simulink model "35 Bus Network Electricity Transmission Model"  (R2023b)
settings: Solver=VariableStepAuto  StartTime=0.0  StopTime=1  RelTol=1e-3
model workspace (MAT data in the model file):
  T_set = 0.0001
  Tp = 5e-05
undefined symbols (not defined in the file): D1, D11, Delta, DiscIntNeverNeededParam
libraries: spsSeriesRLCBranchLib x57, spsLoadFlowBusLib x35, spsThreePhaseSeriesRLCLoadLib x28, spsThreePhaseTransformerTwoWindingsLib x22, spsDistributedParametersLineLib x22, spsGenericPowerSystemStabilizerLib x20, spsThreePhaseVIMeasurementLib x14, spsSynchronousMachinepuStandardLib x10, spsExcitationSystemLib x10, spsHydraulicTurbineandGovernorLib x10, spsFourierLib x8, spsMeanLib x8
(part 6 of 8)

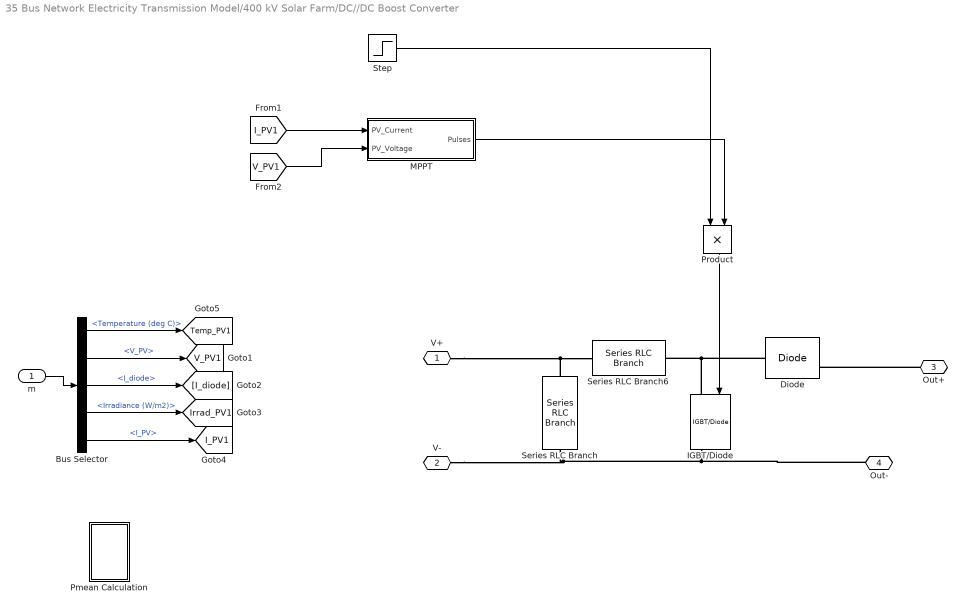
== system 35 Bus Network Electricity Transmission Model/400 kV Solar Farm/DC//DC Boost Converter ==
  m : Inport
  Bus Selector : BusSelector  OutputSignals=Temperature (deg C),V_PV,I_diode,Irradiance (W/m2),I_PV
  Diode : spsDiodeLib/Diode  Ron=0.0001  Lon=0  Vf=0.8  IC=0  UseSnubber=0  Rs=500  Cs=250e-9  Measurements=on
  IGBT/Diode : spsIGBTDiodeLib/IGBT//Diode  Ron=1e-3  Rs=1e5  Cs=inf  Measurements=on
  MPPT : Subsystem  mask{fp=5000, MPPT_time=2e-4, Di=0.62}
      mask prompts: fp "PWM Frequency"; MPPT_time "Time duration for MPPT"; Di "Initialization for Duty Cycle"
  Pmean Calculation : Subsystem
  Product : Product
  Series RLC Branch : spsSeriesRLCBranchLib/Series RLC Branch  LConnTagsString=__new0  RConnTagsString=__new0  BranchType=C  Resistance=1  Inductance=1e-3  SetiL0=off  InitialCurrent=0  Capacitance=1e-4  Setx0=off  InitialVoltage=0  Measurements=None
  Series RLC Branch6 : spsSeriesRLCBranchLib/Series RLC Branch  LConnTagsString=__new0  RConnTagsString=__new0  BranchType=RL  Resistance=0.005  Inductance=5e-3  SetiL0=off  InitialCurrent=0  Capacitance=0  Setx0=off  InitialVoltage=0  Measurements=None
  Step : Step  Time=0.02  SampleTime=0
  V+ : PMIOPort  Side=Left
  V- : PMIOPort  Port=2  Side=Left
  Out+ : PMIOPort  Port=3  Side=Right
  Out- : PMIOPort  Port=4  Side=Right
  tag scope: I_PV1=global, Irrad_PV1=global, Temp_PV1=global, V_PV1=global
  wires:
  [I_PV1] -> MPPT/1(PV_Current)
  Bus Selector/3 -> [I_diode]  "<I_diode>"
  m/1 -> Bus Selector/1
  Bus Selector/5 -> [I_PV1]  "<I_PV>"
  Bus Selector/1 -> [Temp_PV1]  "<Temperature (deg C)>"
  Bus Selector/2 -> [V_PV1]  "<V_PV>"
  [V_PV1] -> MPPT/2(PV_Voltage)
  Step/1 -> Product/1
  MPPT/1(Pulses) -> Product/2
  Product/1 -> IGBT/Diode/1
  Bus Selector/4 -> [Irrad_PV1]  "<Irradiance (W/m2)>"
  connections:
  Series RLC Branch/LConn1 -- V+/RConn1 -- Series RLC Branch6/LConn1
  IGBT/Diode/LConn1 -- Diode/LConn1 -- Series RLC Branch6/RConn1
  IGBT/Diode/RConn1 -- Out-/RConn1 -- V-/RConn1 -- Series RLC Branch/RConn1
  Out+/RConn1 -- Diode/RConn1

== system 35 Bus Network Electricity Transmission Model/400 kV Solar Farm/DC//DC Boost Converter1 ==
  m : Inport
  Bus Selector : BusSelector  OutputSignals=Temperature (deg C),V_PV,I_diode,Irradiance (W/m2),I_PV
  Deblock Converter : Step  Time=0.02  SampleTime=0
  Diode : spsDiodeLib/Diode  Ron=0.0001  Lon=0  Vf=0.8  IC=0  UseSnubber=0  Rs=inf  Cs=inf  Measurements=on
  IGBT/Diode : spsIGBTDiodeLib/IGBT//Diode  Ron=1e-3  Rs=1e5  Cs=inf  Measurements=on
  MPPT : Subsystem  mask{fp=5000, MPPT_time=2e-4, Di=0.62}
      mask prompts: fp "PWM Frequency"; MPPT_time "Time duration for MPPT"; Di "Initialization for Duty Cycle"
  Pmean Calculation : Subsystem
  Product : Product
  Series RLC Branch : spsSeriesRLCBranchLib/Series RLC Branch  LConnTagsString=__new0  RConnTagsString=__new0  BranchType=C  Resistance=1  Inductance=1e-3  SetiL0=off  InitialCurrent=0  Capacitance=1e-4  Setx0=off  InitialVoltage=0  Measurements=None
  Series RLC Branch6 : spsSeriesRLCBranchLib/Series RLC Branch  LConnTagsString=__new0  RConnTagsString=__new0  BranchType=RL  Resistance=0.005  Inductance=5e-3  SetiL0=off  InitialCurrent=0  Capacitance=0  Setx0=off  InitialVoltage=0  Measurements=None
  V+ : PMIOPort  Side=Left
  V- : PMIOPort  Port=2  Side=Left
  Out+ : PMIOPort  Port=3  Side=Right
  Out- : PMIOPort  Port=4  Side=Right
  tag scope: I_PV2=global, Irrad_PV2=global, Temp_PV2=global, V_PV2=global
  wires:
  [I_PV2] -> MPPT/1(PV_Current)
  Bus Selector/3 -> [I_diode]  "<I_diode>"
  m/1 -> Bus Selector/1
  Bus Selector/5 -> [I_PV2]  "<I_PV>"
  Bus Selector/1 -> [Temp_PV2]  "<Temperature (deg C)>"
  Bus Selector/2 -> [V_PV2]  "<V_PV>"
  Bus Selector/4 -> [Irrad_PV2]  "<Irradiance (W/m2)>"
  [V_PV2] -> MPPT/2(PV_Voltage)
  MPPT/1(Pulses) -> Product/1
  Deblock Converter/1 -> Product/2
  Product/1 -> IGBT/Diode/1
  connections:
  Series RLC Branch6/LConn1 -- Series RLC Branch/LConn1 -- V+/RConn1
  IGBT/Diode/LConn1 -- Diode/LConn1 -- Series RLC Branch6/RConn1
  V-/RConn1 -- Series RLC Branch/RConn1 -- IGBT/Diode/RConn1 -- Out-/RConn1
  Out+/RConn1 -- Diode/RConn1

== system 35 Bus Network Electricity Transmission Model/400 kV Solar Farm/DC//DC Boost Converter2 ==
  m : Inport
  Bus Selector : BusSelector  OutputSignals=Temperature (deg C),V_PV,I_diode,Irradiance (W/m2),I_PV
  Diode : spsDiodeLib/Diode  Ron=0.0001  Lon=0  Vf=0.8  IC=0  UseSnubber=0  Rs=inf  Cs=inf  Measurements=on
  IGBT/Diode : spsIGBTDiodeLib/IGBT//Diode  Ron=1e-3  Rs=1e5  Cs=inf  Measurements=on
  MPPT : Subsystem  mask{fp=5000, MPPT_time=2e-4, Di=0.62}
      mask prompts: fp "PWM Frequency"; MPPT_time "Time duration for MPPT"; Di "Initialization for Duty Cycle"
  Pmean Calculation : Subsystem
  Product : Product
  Series RLC Branch : spsSeriesRLCBranchLib/Series RLC Branch  LConnTagsString=__new0  RConnTagsString=__new0  BranchType=C  Resistance=1  Inductance=1e-3  SetiL0=off  InitialCurrent=0  Capacitance=1e-4  Setx0=off  InitialVoltage=0  Measurements=None
  Series RLC Branch6 : spsSeriesRLCBranchLib/Series RLC Branch  LConnTagsString=__new0  RConnTagsString=__new0  BranchType=RL  Resistance=0.005  Inductance=5e-3  SetiL0=off  InitialCurrent=0  Capacitance=0  Setx0=off  InitialVoltage=0  Measurements=None
  Step : Step  Time=0.02  SampleTime=0
  V+ : PMIOPort  Side=Left
  V- : PMIOPort  Port=2  Side=Left
  Out+ : PMIOPort  Port=3  Side=Right
  Out- : PMIOPort  Port=4  Side=Right
  tag scope: I_PV3=global, Irrad_PV3=global, Temp_PV3=global, V_PV3=global
  wires:
  [I_PV3] -> MPPT/1(PV_Current)
  Bus Selector/3 -> [I_diode]  "<I_diode>"
  m/1 -> Bus Selector/1
  Bus Selector/5 -> [I_PV3]  "<I_PV>"
  Bus Selector/1 -> [Temp_PV3]  "<Temperature (deg C)>"
  Bus Selector/2 -> [V_PV3]  "<V_PV>"
  Bus Selector/4 -> [Irrad_PV3]  "<Irradiance (W/m2)>"
  [V_PV3] -> MPPT/2(PV_Voltage)
  Step/1 -> Product/2
  MPPT/1(Pulses) -> Product/1
  Product/1 -> IGBT/Diode/1
  connections:
  Series RLC Branch6/LConn1 -- Series RLC Branch/LConn1 -- V+/RConn1
  IGBT/Diode/LConn1 -- Diode/LConn1 -- Series RLC Branch6/RConn1
  V-/RConn1 -- Series RLC Branch/RConn1 -- IGBT/Diode/RConn1 -- Out-/RConn1
  Out+/RConn1 -- Diode/RConn1

== system 35 Bus Network Electricity Transmission Model/400 kV Solar Farm/DC//DC Boost Converter3 ==
  m : Inport
  Bus Selector : BusSelector  OutputSignals=Temperature (deg C),V_PV,I_diode,Irradiance (W/m2),I_PV
  Diode : spsDiodeLib/Diode  Ron=0.0001  Lon=0  Vf=0.8  IC=0  UseSnubber=0  Rs=inf  Cs=inf  Measurements=on
  IGBT/Diode : spsIGBTDiodeLib/IGBT//Diode  Ron=1e-3  Rs=1e5  Cs=inf  Measurements=on
  MPPT : Subsystem  mask{fp=5000, MPPT_time=2e-4, Di=0.62}
      mask prompts: fp "PWM Frequency"; MPPT_time "Time duration for MPPT"; Di "Initialization for Duty Cycle"
  Pmean Calculation : Subsystem
  Product : Product
  Series RLC Branch : spsSeriesRLCBranchLib/Series RLC Branch  LConnTagsString=__new0  RConnTagsString=__new0  BranchType=C  Resistance=1  Inductance=1e-3  SetiL0=off  InitialCurrent=0  Capacitance=1e-4  Setx0=off  InitialVoltage=0  Measurements=None
  Series RLC Branch6 : spsSeriesRLCBranchLib/Series RLC Branch  LConnTagsString=__new0  RConnTagsString=__new0  BranchType=RL  Resistance=0.005  Inductance=5e-3  SetiL0=off  InitialCurrent=0  Capacitance=0  Setx0=off  InitialVoltage=0  Measurements=None
  Step : Step  Time=0.02  SampleTime=0
  V+ : PMIOPort  Side=Left
  V- : PMIOPort  Port=2  Side=Left
  Out+ : PMIOPort  Port=3  Side=Right
  Out- : PMIOPort  Port=4  Side=Right
  tag scope: I_PV4=global, Irrad_PV4=global, Temp_PV4=global, V_PV4=global
  wires:
  [I_PV4] -> MPPT/1(PV_Current)
  Bus Selector/3 -> [I_diode]  "<I_diode>"
  m/1 -> Bus Selector/1
  Bus Selector/5 -> [I_PV4]  "<I_PV>"
  Bus Selector/1 -> [Temp_PV4]  "<Temperature (deg C)>"
  Bus Selector/2 -> [V_PV4]  "<V_PV>"
  [V_PV4] -> MPPT/2(PV_Voltage)
  Step/1 -> Product/2
  MPPT/1(Pulses) -> Product/1
  Product/1 -> IGBT/Diode/1
  Bus Selector/4 -> [Irrad_PV4]  "<Irradiance (W/m2)>"
  connections:
  Series RLC Branch6/LConn1 -- Series RLC Branch/LConn1 -- V+/RConn1
  IGBT/Diode/LConn1 -- Diode/LConn1 -- Series RLC Branch6/RConn1
  V-/RConn1 -- Series RLC Branch/RConn1 -- IGBT/Diode/RConn1 -- Out-/RConn1
  Out+/RConn1 -- Diode/RConn1

== system 35 Bus Network Electricity Transmission Model/400 kV Solar Farm/VSC Control ==
  Vabc_prim : Inport  PortDimensions=3
  Iabc_prim : Inport  Port=2  PortDimensions=3
  Vdc_mes : Inport  Port=3  PortDimensions=1
  Current Regulator : Subsystem
  Iq_ref : Constant  Value=0
  Mux : Mux  Inputs=2
  PLL & Measurements : Subsystem
  PWM Generator (3-Level) : spsPWMGenerator3LevelLib/PWM Generator (3-Level)  ModulatorType=Three-phase bridge (12 pulses)  ModulatorMode=Unsynchronized  nF=27  Fc=33*60  ModulatingSignals=off  m=0.8  Freq=60  Phase=0  Ts=5e-5
  Uabc_ref Generation max (m) = 1 : Subsystem
  Unit Delay : UnitDelay  SampleTime=T_set  HasFrameUpgradeWarning=on
  VDC Regulator : Subsystem
  Vdc_ref1 : Constant  Value=Vdc_ref
  Pulses : Outport  VectorParamsAs1DForOutWhenUnconnected=off
  wires:
  VDC Regulator/1(Id_ref) -> Mux/1
  PLL & Measurements/1(wt) -> Uabc_ref Generation max (m) = 1/1(wt)
  Current Regulator/1(VdVq_conv) -> Uabc_ref Generation max (m) = 1/2(VdVq_conv)
  Iq_ref/1 -> Mux/2
  Mux/1 -> Current Regulator/3(IdIq_ref)
  PLL & Measurements/3(IdIq_prim) -> Current Regulator/2(IdIq_mes)
  PLL & Measurements/2(VdVq_prim) -> Current Regulator/1(VdVq_mes)
  Vdc_mes/1 -> VDC Regulator/1(Vdc_mes)
  Vabc_prim/1 -> PLL & Measurements/1(Vabc_prim)
  Iabc_prim/1 -> PLL & Measurements/2(Iabc_prim)
  Unit Delay/1 -> PWM Generator (3-Level)/1
  PWM Generator (3-Level)/1 -> Pulses/1
  Uabc_ref Generation max (m) = 1/1(Uabc_ref) -> Unit Delay/1
  Vdc_ref1/1 -> VDC Regulator/2(Vdc_ref)

== system 35 Bus Network Electricity Transmission Model/Home Network Load （with circuit breaker)/Circuit Breaker ==
  "Reset " : Inport
  Abs : Abs  SaturateOnIntegerOverflow=off
  Current Measurement1 : spsCurrentMeasurementLib/Current Measurement  PhasorSimulation=off  OutputType=Complex  PSBequivalent=0
  Data Type Conversion : DataTypeConversion  OutDataTypeStr=boolean  SaturateOnIntegerOverflow=off  RndMeth=Floor
  Data Type Conversion1 : DataTypeConversion  OutDataTypeStr=double  SaturateOnIntegerOverflow=off  RndMeth=Floor
  Hit Crossing : HitCross
  Ideal Switch : spsIdealSwitchLib/Ideal Switch  Ron=0.01  Lon=0  IC=0  Rs=1e5  Cs=inf  Measurements=on
  Logical Operator : Logic  AllPortsSameDT=off  OutDataTypeStr=boolean
  Relational Operator : RelationalOperator  Operator=<=  OutDataTypeStr=boolean  RndMeth=Simplest  InputSameDT=off
  S-R Flip-Flop : simulink_extras/Flip Flops/S-R Flip-Flop  initial_condition=0
  S-R Flip-Flop1 : simulink_extras/Flip Flops/S-R Flip-Flop  initial_condition=0
  Static Trip Current : Constant  Value=110
  Terminator : Terminator
  Terminator1 : Terminator
  Terminator2 : Terminator
  Transfer Fcn : TransferFcn  Denominator=[0.001 1]
  Connection Port1 : PMIOPort  Side=Left
  Connection Port : PMIOPort  Port=2  Side=Right
  wires:
  Logical Operator/1 -> S-R Flip-Flop1/2
  Current Measurement1/1 -> Hit Crossing/1, Abs/1
  Hit Crossing/1 -> Logical Operator/2
  Transfer Fcn/1 -> Relational Operator/1
  S-R Flip-Flop1/2 -> Terminator1/1
  Ideal Switch/1 -> Terminator2/1
  S-R Flip-Flop/1 -> Logical Operator/1
  Abs/1 -> Transfer Fcn/1
  "Reset "/1 -> Data Type Conversion/1
  S-R Flip-Flop1/1 -> Data Type Conversion1/1
  Relational Operator/1 -> S-R Flip-Flop/1
  Data Type Conversion/1 -> S-R Flip-Flop/2, S-R Flip-Flop1/1
  S-R Flip-Flop/2 -> Terminator/1
  Data Type Conversion1/1 -> Ideal Switch/1
  Static Trip Current/1 -> Relational Operator/2
  connections:
  Connection Port1/RConn1 -- Ideal Switch/LConn1
  Current Measurement1/LConn1 -- Ideal Switch/RConn1
  Connection Port/RConn1 -- Current Measurement1/RConn1

== system 35 Bus Network Electricity Transmission Model/North Network/Cs BMW- MPP8 ==
  Series RLC Branch : spsSeriesRLCBranchLib/Series RLC Branch  LConnTagsString=__new0  RConnTagsString=__new0  BranchType=C  Resistance=1  Inductance=1e-3  SetiL0=off  InitialCurrent=0  Capacitance=0.00049736  Setx0=off  InitialVoltage=0  Measurements=None
  Series RLC Branch1 : spsSeriesRLCBranchLib/Series RLC Branch  LConnTagsString=__new0  RConnTagsString=__new0  BranchType=C  Resistance=1  Inductance=1e-3  SetiL0=off  InitialCurrent=0  Capacitance=0.00049736  Setx0=off  InitialVoltage=0  Measurements=None
  Series RLC Branch2 : spsSeriesRLCBranchLib/Series RLC Branch  LConnTagsString=__new0  RConnTagsString=__new0  BranchType=C  Resistance=1  Inductance=1e-3  SetiL0=off  InitialCurrent=0  Capacitance=0.00049736  Setx0=off  InitialVoltage=0  Measurements=None
  A : PMIOPort  Side=Left
  A1 : PMIOPort  Port=2  Side=Right
  B : PMIOPort  Port=3  Side=Left
  B1 : PMIOPort  Port=4  Side=Right
  C : PMIOPort  Port=5  Side=Left
  C1 : PMIOPort  Port=6  Side=Right
  connections:
  A1/RConn1 -- Series RLC Branch/RConn1
  B1/RConn1 -- Series RLC Branch1/RConn1
  A/RConn1 -- Series RLC Branch/LConn1
  C/RConn1 -- Series RLC Branch2/LConn1
  B/RConn1 -- Series RLC Branch1/LConn1
  C1/RConn1 -- Series RLC Branch2/RConn1

== system 35 Bus Network Electricity Transmission Model/North Network/Cs BMWN ==
  Series RLC Branch : spsSeriesRLCBranchLib/Series RLC Branch  LConnTagsString=__new0  RConnTagsString=__new0  BranchType=C  Resistance=1  Inductance=1e-3  SetiL0=off  InitialCurrent=0  Capacitance=0.00049736  Setx0=off  InitialVoltage=0  Measurements=None
  Series RLC Branch1 : spsSeriesRLCBranchLib/Series RLC Branch  LConnTagsString=__new0  RConnTagsString=__new0  BranchType=C  Resistance=1  Inductance=1e-3  SetiL0=off  InitialCurrent=0  Capacitance=0.00049736  Setx0=off  InitialVoltage=0  Measurements=None
  Series RLC Branch2 : spsSeriesRLCBranchLib/Series RLC Branch  LConnTagsString=__new0  RConnTagsString=__new0  BranchType=C  Resistance=1  Inductance=1e-3  SetiL0=off  InitialCurrent=0  Capacitance=0.00049736  Setx0=off  InitialVoltage=0  Measurements=None
  A : PMIOPort  Side=Left
  A1 : PMIOPort  Port=2  Side=Right
  B : PMIOPort  Port=3  Side=Left
  B1 : PMIOPort  Port=4  Side=Right
  C : PMIOPort  Port=5  Side=Left
  C1 : PMIOPort  Port=6  Side=Right
  connections:
  A1/RConn1 -- Series RLC Branch/RConn1
  B1/RConn1 -- Series RLC Branch1/RConn1
  A/RConn1 -- Series RLC Branch/LConn1
  C/RConn1 -- Series RLC Branch2/LConn1
  B/RConn1 -- Series RLC Branch1/LConn1
  C1/RConn1 -- Series RLC Branch2/RConn1

== system 35 Bus Network Electricity Transmission Model/North Network/Cs FER ==
  Series RLC Branch : spsSeriesRLCBranchLib/Series RLC Branch  LConnTagsString=__new0  RConnTagsString=__new0  BranchType=C  Resistance=1  Inductance=1e-3  SetiL0=off  InitialCurrent=0  Capacitance=0.00049736  Setx0=off  InitialVoltage=0  Measurements=None
  Series RLC Branch1 : spsSeriesRLCBranchLib/Series RLC Branch  LConnTagsString=__new0  RConnTagsString=__new0  BranchType=C  Resistance=1  Inductance=1e-3  SetiL0=off  InitialCurrent=0  Capacitance=0.00049736  Setx0=off  InitialVoltage=0  Measurements=None
  Series RLC Branch2 : spsSeriesRLCBranchLib/Series RLC Branch  LConnTagsString=__new0  RConnTagsString=__new0  BranchType=C  Resistance=1  Inductance=1e-3  SetiL0=off  InitialCurrent=0  Capacitance=0.00049736  Setx0=off  InitialVoltage=0  Measurements=None
  A : PMIOPort  Side=Left
  A1 : PMIOPort  Port=2  Side=Right
  B : PMIOPort  Port=3  Side=Left
  B1 : PMIOPort  Port=4  Side=Right
  C : PMIOPort  Port=5  Side=Left
  C1 : PMIOPort  Port=6  Side=Right
  connections:
  A1/RConn1 -- Series RLC Branch/RConn1
  B1/RConn1 -- Series RLC Branch1/RConn1
  A/RConn1 -- Series RLC Branch/LConn1
  C/RConn1 -- Series RLC Branch2/LConn1
  B/RConn1 -- Series RLC Branch1/LConn1
  C1/RConn1 -- Series RLC Branch2/RConn1

== system 35 Bus Network Electricity Transmission Model/North Network/Cs LTNN ==
  Series RLC Branch : spsSeriesRLCBranchLib/Series RLC Branch  LConnTagsString=__new0  RConnTagsString=__new0  BranchType=C  Resistance=1  Inductance=1e-3  SetiL0=off  InitialCurrent=0  Capacitance=0.00049736  Setx0=off  InitialVoltage=0  Measurements=None
  Series RLC Branch1 : spsSeriesRLCBranchLib/Series RLC Branch  LConnTagsString=__new0  RConnTagsString=__new0  BranchType=C  Resistance=1  Inductance=1e-3  SetiL0=off  InitialCurrent=0  Capacitance=0.00049736  Setx0=off  InitialVoltage=0  Measurements=None
  Series RLC Branch2 : spsSeriesRLCBranchLib/Series RLC Branch  LConnTagsString=__new0  RConnTagsString=__new0  BranchType=C  Resistance=1  Inductance=1e-3  SetiL0=off  InitialCurrent=0  Capacitance=0.00049736  Setx0=off  InitialVoltage=0  Measurements=None
  A : PMIOPort  Side=Left
  A1 : PMIOPort  Port=2  Side=Right
  B : PMIOPort  Port=3  Side=Left
  B1 : PMIOPort  Port=4  Side=Right
  C : PMIOPort  Port=5  Side=Left
  C1 : PMIOPort  Port=6  Side=Right
  connections:
  A1/RConn1 -- Series RLC Branch/RConn1
  B1/RConn1 -- Series RLC Branch1/RConn1
  A/RConn1 -- Series RLC Branch/LConn1
  C/RConn1 -- Series RLC Branch2/LConn1
  B/RConn1 -- Series RLC Branch1/LConn1
  C1/RConn1 -- Series RLC Branch2/RConn1

== system 35 Bus Network Electricity Transmission Model/North Network/Cs ORED ==
  Series RLC Branch : spsSeriesRLCBranchLib/Series RLC Branch  LConnTagsString=__new0  RConnTagsString=__new0  BranchType=C  Resistance=1  Inductance=1e-3  SetiL0=off  InitialCurrent=0  Capacitance=0.00049736  Setx0=off  InitialVoltage=0  Measurements=None
  Series RLC Branch1 : spsSeriesRLCBranchLib/Series RLC Branch  LConnTagsString=__new0  RConnTagsString=__new0  BranchType=C  Resistance=1  Inductance=1e-3  SetiL0=off  InitialCurrent=0  Capacitance=0.00049736  Setx0=off  InitialVoltage=0  Measurements=None
  Series RLC Branch2 : spsSeriesRLCBranchLib/Series RLC Branch  LConnTagsString=__new0  RConnTagsString=__new0  BranchType=C  Resistance=1  Inductance=1e-3  SetiL0=off  InitialCurrent=0  Capacitance=0.00049736  Setx0=off  InitialVoltage=0  Measurements=None
  A : PMIOPort  Side=Left
  A1 : PMIOPort  Port=2  Side=Right
  B : PMIOPort  Port=3  Side=Left
  B1 : PMIOPort  Port=4  Side=Right
  C : PMIOPort  Port=5  Side=Left
  C1 : PMIOPort  Port=6  Side=Right
  connections:
  A1/RConn1 -- Series RLC Branch/RConn1
  B1/RConn1 -- Series RLC Branch1/RConn1
  A/RConn1 -- Series RLC Branch/LConn1
  C/RConn1 -- Series RLC Branch2/LConn1
  B/RConn1 -- Series RLC Branch1/LConn1
  C1/RConn1 -- Series RLC Branch2/RConn1

== system 35 Bus Network Electricity Transmission Model/North Network/Regulators 7 ==
  m : Inport
  Bus Selector : BusSelector  OutputSignals="dq0 components.Stator voltage  vq (pu),dq0 components.Stator voltage  vd (pu),Mechanical.Rotor speed  wm  (pu),Output active power   Peo (pu)"
  Constant : Constant  Value=0.8148
  Constant1 : Constant
  Math Function : Math  Operator=hypot
  Turbine and Excitation Regulators : Subsystem
  Pm : Outport
  Vf : Outport  Port=2
  tag scope: Vm7=global, w7=global
  wires:
  Bus Selector/4 -> Turbine and Excitation Regulators/3(Pe 0)  "<Output active power   Peo (pu)>"
  Constant1/1 -> Turbine and Excitation Regulators/4(Vref)
  Bus Selector/3 -> [w7], Turbine and Excitation Regulators/2(w)  "<Rotor speed  wm  (pu)>"
  Turbine and Excitation Regulators/1(Pm) -> Pm/1
  m/1 -> Bus Selector/1
  Turbine and Excitation Regulators/2(Vf) -> Vf/1
  Bus Selector/1 -> Math Function/1  "<Stator voltage  vq (pu)>"
  Math Function/1 -> [Vm7], Turbine and Excitation Regulators/5(Vm)
  Bus Selector/2 -> Math Function/2  "<Stator voltage  vd (pu)>"
  Constant/1 -> Turbine and Excitation Regulators/1(pref)

== system 35 Bus Network Electricity Transmission Model/North Network/Regulators 8 ==
  m : Inport
  Bus Selector : BusSelector  OutputSignals="dq0 components.Stator voltage  vq (pu),dq0 components.Stator voltage  vd (pu),Mechanical.Rotor speed  wm  (pu),Output active power   Peo (pu)"
  Constant : Constant  Value=0.935
  Constant1 : Constant
  Math Function : Math  Operator=hypot
  Turbine and Excitation Regulators : Subsystem
  Pm : Outport
  Vf : Outport  Port=2
  tag scope: Vm8=global, w8=global
  wires:
  Bus Selector/4 -> Turbine and Excitation Regulators/3(Pe 0)  "<Output active power   Peo (pu)>"
  Constant1/1 -> Turbine and Excitation Regulators/4(Vref)
  Bus Selector/3 -> [w8], Turbine and Excitation Regulators/2(w)  "<Rotor speed  wm  (pu)>"
  Turbine and Excitation Regulators/1(Pm) -> Pm/1
  m/1 -> Bus Selector/1
  Turbine and Excitation Regulators/2(Vf) -> Vf/1
  Bus Selector/1 -> Math Function/1  "<Stator voltage  vq (pu)>"
  Math Function/1 -> [Vm8], Turbine and Excitation Regulators/5(Vm)
  Bus Selector/2 -> Math Function/2  "<Stator voltage  vd (pu)>"
  Constant/1 -> Turbine and Excitation Regulators/1(pref)

== system 35 Bus Network Electricity Transmission Model/North Network/Regulators 9 ==
  m : Inport
  Bus Selector : BusSelector  OutputSignals="dq0 components.Stator voltage  vq (pu),dq0 components.Stator voltage  vd (pu),Mechanical.Rotor speed  wm  (pu),Output active power   Peo (pu)"
  Constant : Constant  Value=0.854
  Constant1 : Constant
  Math Function : Math  Operator=hypot
  Turbine and Excitation Regulators : Subsystem
  Pm : Outport
  Vf : Outport  Port=2
  tag scope: Vm9=global, w9=global
  wires:
  Bus Selector/4 -> Turbine and Excitation Regulators/3(Pe 0)  "<Output active power   Peo (pu)>"
  Constant1/1 -> Turbine and Excitation Regulators/4(Vref)
  Bus Selector/3 -> [w9], Turbine and Excitation Regulators/2(w)  "<Rotor speed  wm  (pu)>"
  Turbine and Excitation Regulators/1(Pm) -> Pm/1
  m/1 -> Bus Selector/1
  Turbine and Excitation Regulators/2(Vf) -> Vf/1
  Bus Selector/1 -> Math Function/1  "<Stator voltage  vq (pu)>"
  Math Function/1 -> [Vm9], Turbine and Excitation Regulators/5(Vm)
  Bus Selector/2 -> Math Function/2  "<Stator voltage  vd (pu)>"
  Constant/1 -> Turbine and Excitation Regulators/1(pref)

== system 35 Bus Network Electricity Transmission Model/Regulators 10/Turbine and Excitation Regulators ==
  pref : Inport
  w : Inport  Port=2
  Pe 0 : Inport  Port=3
  Vref : Inport  Port=4
  Vm : Inport  Port=5
  Add : Sum  Inputs=+-
  Complex to Real-Imag : ComplexToRealImag
  Excitation System : spsExcitationSystemLib/Excitation System  tr=20e-3  reg=[ 300, 0.001 ]  exc=[ 1, 0 ]  tgr=[ 0, 0 ]  damp=[ 0.001, 0.1 ]  sat=[ 0, 0 ]  lim=[ -11.5, 11.5, 0 ]  v0="[1.0  1.28]"
      settings: LibrarySourceBlock=sps_lib/Electrical Machines/Synchronous Machine Control/Excitation System
  Hydraulic Turbine and Governor : spsHydraulicTurbineandGovernorLib/Hydraulic Turbine and Governor  sm="[ 10/3  0.07 ]"  gate="[  0.01  0.97518  -0.1  0.1 ]"  reg="[  0.05  1.163  0.105  0  0.01  ]"  hyd="[  0  2.67  ]"  dref=0  po=0.7516
      settings: LibrarySourceBlock=|
      | sps_lib/Electrical Machines/Synchronous Machine Control/Hydraulic Turbine
      | and Governor
  Stabilitator : Subsystem
  Terminator : Terminator
  wref : Constant
  wref1 : Constant
  Pm : Outport
  Vf : Outport  Port=2
  wires:
  pref/1 -> Hydraulic Turbine and Governor/2
  Complex to Real-Imag/2 -> Excitation System/3
  wref/1 -> Hydraulic Turbine and Governor/1
  Add/1 -> Stabilitator/3(dw), Hydraulic Turbine and Governor/5
  Vm/1 -> Complex to Real-Imag/1
  Pe 0/1 -> Stabilitator/2(Pe), Hydraulic Turbine and Governor/4
  Hydraulic Turbine and Governor/2 -> Terminator/1
  Stabilitator/1(Out1) -> Excitation System/4
  w/1 -> Add/1, Hydraulic Turbine and Governor/3
  Excitation System/1 -> Vf/1
  Hydraulic Turbine and Governor/1 -> Pm/1, Stabilitator/1(Pm)
  Vref/1 -> Excitation System/1
  wref1/1 -> Add/2
  Complex to Real-Imag/1 -> Excitation System/2

== system 35 Bus Network Electricity Transmission Model/South Network/Cs AND ==
  Series RLC Branch : spsSeriesRLCBranchLib/Series RLC Branch  LConnTagsString=__new0  RConnTagsString=__new0  BranchType=C  Resistance=1  Inductance=1e-3  SetiL0=off  InitialCurrent=0  Capacitance=0.00049736  Setx0=off  InitialVoltage=0  Measurements=None
  Series RLC Branch1 : spsSeriesRLCBranchLib/Series RLC Branch  LConnTagsString=__new0  RConnTagsString=__new0  BranchType=C  Resistance=1  Inductance=1e-3  SetiL0=off  InitialCurrent=0  Capacitance=0.00049736  Setx0=off  InitialVoltage=0  Measurements=None
  Series RLC Branch2 : spsSeriesRLCBranchLib/Series RLC Branch  LConnTagsString=__new0  RConnTagsString=__new0  BranchType=C  Resistance=1  Inductance=1e-3  SetiL0=off  InitialCurrent=0  Capacitance=0.00049736  Setx0=off  InitialVoltage=0  Measurements=None
  A : PMIOPort  Side=Left
  A1 : PMIOPort  Port=2  Side=Right
  B : PMIOPort  Port=3  Side=Left
  B1 : PMIOPort  Port=4  Side=Right
  C : PMIOPort  Port=5  Side=Left
  C1 : PMIOPort  Port=6  Side=Right
  connections:
  A1/RConn1 -- Series RLC Branch/RConn1
  B1/RConn1 -- Series RLC Branch1/RConn1
  A/RConn1 -- Series RLC Branch/LConn1
  C/RConn1 -- Series RLC Branch2/LConn1
  B/RConn1 -- Series RLC Branch1/LConn1
  C1/RConn1 -- Series RLC Branch2/RConn1

== system 35 Bus Network Electricity Transmission Model/South Network/Cs CLPN ==
  Series RLC Branch : spsSeriesRLCBranchLib/Series RLC Branch  LConnTagsString=__new0  RConnTagsString=__new0  BranchType=C  Resistance=1  Inductance=1e-3  SetiL0=off  InitialCurrent=0  Capacitance=0.00049736  Setx0=off  InitialVoltage=0  Measurements=None
  Series RLC Branch1 : spsSeriesRLCBranchLib/Series RLC Branch  LConnTagsString=__new0  RConnTagsString=__new0  BranchType=C  Resistance=1  Inductance=1e-3  SetiL0=off  InitialCurrent=0  Capacitance=0.00049736  Setx0=off  InitialVoltage=0  Measurements=None
  Series RLC Branch2 : spsSeriesRLCBranchLib/Series RLC Branch  LConnTagsString=__new0  RConnTagsString=__new0  BranchType=C  Resistance=1  Inductance=1e-3  SetiL0=off  InitialCurrent=0  Capacitance=0.00049736  Setx0=off  InitialVoltage=0  Measurements=None
  A : PMIOPort  Side=Left
  A1 : PMIOPort  Port=2  Side=Right
  B : PMIOPort  Port=3  Side=Left
  B1 : PMIOPort  Port=4  Side=Right
  C : PMIOPort  Port=5  Side=Left
  C1 : PMIOPort  Port=6  Side=Right
  connections:
  A1/RConn1 -- Series RLC Branch/RConn1
  B1/RConn1 -- Series RLC Branch1/RConn1
  A/RConn1 -- Series RLC Branch/LConn1
  C/RConn1 -- Series RLC Branch2/LConn1
  B/RConn1 -- Series RLC Branch1/LConn1
  C1/RConn1 -- Series RLC Branch2/RConn1

== system 35 Bus Network Electricity Transmission Model/South Network/Cs CLPS ==
  Series RLC Branch : spsSeriesRLCBranchLib/Series RLC Branch  LConnTagsString=__new0  RConnTagsString=__new0  BranchType=C  Resistance=1  Inductance=1e-3  SetiL0=off  InitialCurrent=0  Capacitance=0.00049736  Setx0=off  InitialVoltage=0  Measurements=None
  Series RLC Branch1 : spsSeriesRLCBranchLib/Series RLC Branch  LConnTagsString=__new0  RConnTagsString=__new0  BranchType=C  Resistance=1  Inductance=1e-3  SetiL0=off  InitialCurrent=0  Capacitance=0.00049736  Setx0=off  InitialVoltage=0  Measurements=None
  Series RLC Branch2 : spsSeriesRLCBranchLib/Series RLC Branch  LConnTagsString=__new0  RConnTagsString=__new0  BranchType=C  Resistance=1  Inductance=1e-3  SetiL0=off  InitialCurrent=0  Capacitance=0.00049736  Setx0=off  InitialVoltage=0  Measurements=None
  A : PMIOPort  Side=Left
  A1 : PMIOPort  Port=2  Side=Right
  B : PMIOPort  Port=3  Side=Left
  B1 : PMIOPort  Port=4  Side=Right
  C : PMIOPort  Port=5  Side=Left
  C1 : PMIOPort  Port=6  Side=Right
  connections:
  A1/RConn1 -- Series RLC Branch/RConn1
  B1/RConn1 -- Series RLC Branch1/RConn1
  A/RConn1 -- Series RLC Branch/LConn1
  C/RConn1 -- Series RLC Branch2/LConn1
  B/RConn1 -- Series RLC Branch1/LConn1
  C1/RConn1 -- Series RLC Branch2/RConn1

== system 35 Bus Network Electricity Transmission Model/South Network/Cs CSGN ==
  Series RLC Branch : spsSeriesRLCBranchLib/Series RLC Branch  LConnTagsString=__new0  RConnTagsString=__new0  BranchType=C  Resistance=1  Inductance=1e-3  SetiL0=off  InitialCurrent=0  Capacitance=0.00049736  Setx0=off  InitialVoltage=0  Measurements=None
  Series RLC Branch1 : spsSeriesRLCBranchLib/Series RLC Branch  LConnTagsString=__new0  RConnTagsString=__new0  BranchType=C  Resistance=1  Inductance=1e-3  SetiL0=off  InitialCurrent=0  Capacitance=0.00049736  Setx0=off  InitialVoltage=0  Measurements=None
  Series RLC Branch2 : spsSeriesRLCBranchLib/Series RLC Branch  LConnTagsString=__new0  RConnTagsString=__new0  BranchType=C  Resistance=1  Inductance=1e-3  SetiL0=off  InitialCurrent=0  Capacitance=0.00049736  Setx0=off  InitialVoltage=0  Measurements=None
  A : PMIOPort  Side=Left
  A1 : PMIOPort  Port=2  Side=Right
  B : PMIOPort  Port=3  Side=Left
  B1 : PMIOPort  Port=4  Side=Right
  C : PMIOPort  Port=5  Side=Left
  C1 : PMIOPort  Port=6  Side=Right
  connections:
  A1/RConn1 -- Series RLC Branch/RConn1
  B1/RConn1 -- Series RLC Branch1/RConn1
  A/RConn1 -- Series RLC Branch/LConn1
  C/RConn1 -- Series RLC Branch2/LConn1
  B/RConn1 -- Series RLC Branch1/LConn1
  C1/RConn1 -- Series RLC Branch2/RConn1

== system 35 Bus Network Electricity Transmission Model/South Network/Cs MPP1D ==
  Series RLC Branch : spsSeriesRLCBranchLib/Series RLC Branch  LConnTagsString=__new0  RConnTagsString=__new0  BranchType=C  Resistance=1  Inductance=1e-3  SetiL0=off  InitialCurrent=0  Capacitance=0.00049736  Setx0=off  InitialVoltage=0  Measurements=None
  Series RLC Branch1 : spsSeriesRLCBranchLib/Series RLC Branch  LConnTagsString=__new0  RConnTagsString=__new0  BranchType=C  Resistance=1  Inductance=1e-3  SetiL0=off  InitialCurrent=0  Capacitance=0.00049736  Setx0=off  InitialVoltage=0  Measurements=None
  Series RLC Branch2 : spsSeriesRLCBranchLib/Series RLC Branch  LConnTagsString=__new0  RConnTagsString=__new0  BranchType=C  Resistance=1  Inductance=1e-3  SetiL0=off  InitialCurrent=0  Capacitance=0.00049736  Setx0=off  InitialVoltage=0  Measurements=None
  A : PMIOPort  Side=Left
  A1 : PMIOPort  Port=2  Side=Right
  B : PMIOPort  Port=3  Side=Left
  B1 : PMIOPort  Port=4  Side=Right
  C : PMIOPort  Port=5  Side=Left
  C1 : PMIOPort  Port=6  Side=Right
  connections:
  A1/RConn1 -- Series RLC Branch/RConn1
  B1/RConn1 -- Series RLC Branch1/RConn1
  A/RConn1 -- Series RLC Branch/LConn1
  C/RConn1 -- Series RLC Branch2/LConn1
  B/RConn1 -- Series RLC Branch1/LConn1
  C1/RConn1 -- Series RLC Branch2/RConn1

== system 35 Bus Network Electricity Transmission Model/South Network/Cs PNSM ==
  Series RLC Branch : spsSeriesRLCBranchLib/Series RLC Branch  LConnTagsString=__new0  RConnTagsString=__new0  BranchType=C  Resistance=1  Inductance=1e-3  SetiL0=off  InitialCurrent=0  Capacitance=0.00049736  Setx0=off  InitialVoltage=0  Measurements=None
  Series RLC Branch1 : spsSeriesRLCBranchLib/Series RLC Branch  LConnTagsString=__new0  RConnTagsString=__new0  BranchType=C  Resistance=1  Inductance=1e-3  SetiL0=off  InitialCurrent=0  Capacitance=0.00049736  Setx0=off  InitialVoltage=0  Measurements=None
  Series RLC Branch2 : spsSeriesRLCBranchLib/Series RLC Branch  LConnTagsString=__new0  RConnTagsString=__new0  BranchType=C  Resistance=1  Inductance=1e-3  SetiL0=off  InitialCurrent=0  Capacitance=0.00049736  Setx0=off  InitialVoltage=0  Measurements=None
  A : PMIOPort  Side=Left
  A1 : PMIOPort  Port=2  Side=Right
  B : PMIOPort  Port=3  Side=Left
  B1 : PMIOPort  Port=4  Side=Right
  C : PMIOPort  Port=5  Side=Left
  C1 : PMIOPort  Port=6  Side=Right
  connections:
  A1/RConn1 -- Series RLC Branch/RConn1
  B1/RConn1 -- Series RLC Branch1/RConn1
  A/RConn1 -- Series RLC Branch/LConn1
  C/RConn1 -- Series RLC Branch2/LConn1
  B/RConn1 -- Series RLC Branch1/LConn1
  C1/RConn1 -- Series RLC Branch2/RConn1

== system 35 Bus Network Electricity Transmission Model/South Network/Cs PNSN ==
  Series RLC Branch : spsSeriesRLCBranchLib/Series RLC Branch  LConnTagsString=__new0  RConnTagsString=__new0  BranchType=C  Resistance=1  Inductance=1e-3  SetiL0=off  InitialCurrent=0  Capacitance=0.00049736  Setx0=off  InitialVoltage=0  Measurements=None
  Series RLC Branch1 : spsSeriesRLCBranchLib/Series RLC Branch  LConnTagsString=__new0  RConnTagsString=__new0  BranchType=C  Resistance=1  Inductance=1e-3  SetiL0=off  InitialCurrent=0  Capacitance=0.00049736  Setx0=off  InitialVoltage=0  Measurements=None
  Series RLC Branch2 : spsSeriesRLCBranchLib/Series RLC Branch  LConnTagsString=__new0  RConnTagsString=__new0  BranchType=C  Resistance=1  Inductance=1e-3  SetiL0=off  InitialCurrent=0  Capacitance=0.00049736  Setx0=off  InitialVoltage=0  Measurements=None
  A : PMIOPort  Side=Left
  A1 : PMIOPort  Port=2  Side=Right
  B : PMIOPort  Port=3  Side=Left
  B1 : PMIOPort  Port=4  Side=Right
  C : PMIOPort  Port=5  Side=Left
  C1 : PMIOPort  Port=6  Side=Right
  connections:
  A1/RConn1 -- Series RLC Branch/RConn1
  B1/RConn1 -- Series RLC Branch1/RConn1
  A/RConn1 -- Series RLC Branch/LConn1
  C/RConn1 -- Series RLC Branch2/LConn1
  B/RConn1 -- Series RLC Branch1/LConn1
  C1/RConn1 -- Series RLC Branch2/RConn1

== system 35 Bus Network Electricity Transmission Model/South Network/Cs SATS ==
  Series RLC Branch : spsSeriesRLCBranchLib/Series RLC Branch  LConnTagsString=__new0  RConnTagsString=__new0  BranchType=C  Resistance=1  Inductance=1e-3  SetiL0=off  InitialCurrent=0  Capacitance=0.00049736  Setx0=off  InitialVoltage=0  Measurements=None
  Series RLC Branch1 : spsSeriesRLCBranchLib/Series RLC Branch  LConnTagsString=__new0  RConnTagsString=__new0  BranchType=C  Resistance=1  Inductance=1e-3  SetiL0=off  InitialCurrent=0  Capacitance=0.00049736  Setx0=off  InitialVoltage=0  Measurements=None
  Series RLC Branch2 : spsSeriesRLCBranchLib/Series RLC Branch  LConnTagsString=__new0  RConnTagsString=__new0  BranchType=C  Resistance=1  Inductance=1e-3  SetiL0=off  InitialCurrent=0  Capacitance=0.00049736  Setx0=off  InitialVoltage=0  Measurements=None
  A : PMIOPort  Side=Left
  A1 : PMIOPort  Port=2  Side=Right
  B : PMIOPort  Port=3  Side=Left
  B1 : PMIOPort  Port=4  Side=Right
  C : PMIOPort  Port=5  Side=Left
  C1 : PMIOPort  Port=6  Side=Right
  connections:
  A1/RConn1 -- Series RLC Branch/RConn1
  B1/RConn1 -- Series RLC Branch1/RConn1
  A/RConn1 -- Series RLC Branch/LConn1
  C/RConn1 -- Series RLC Branch2/LConn1
  B/RConn1 -- Series RLC Branch1/LConn1
  C1/RConn1 -- Series RLC Branch2/RConn1

== system 35 Bus Network Electricity Transmission Model/South Network/Regulators 1 ==
  m : Inport
  Bus Selector : BusSelector  OutputSignals="dq0 components.Stator voltage  vq (pu),dq0 components.Stator voltage  vd (pu),Mechanical.Rotor speed  wm  (pu),Output active power   Peo (pu)"
  Constant : Constant  Value=0.811
  Constant1 : Constant
  Math Function : Math  Operator=hypot
  Turbine and Excitation Regulators : Subsystem
  Pm : Outport
  Vf : Outport  Port=2
  tag scope: Vm1=global, w1=global
  wires:
  Constant1/1 -> Turbine and Excitation Regulators/4(Vref)
  Turbine and Excitation Regulators/1(Pm) -> Pm/1
  m/1 -> Bus Selector/1
  Turbine and Excitation Regulators/2(Vf) -> Vf/1
  Math Function/1 -> [Vm1], Turbine and Excitation Regulators/5(Vm)
  Constant/1 -> Turbine and Excitation Regulators/1(pref)
  Bus Selector/1 -> Math Function/1  "<Stator voltage  vq (pu)>"
  Bus Selector/2 -> Math Function/2  "<Stator voltage  vd (pu)>"
  Bus Selector/4 -> Turbine and Excitation Regulators/3(Pe 0)  "<Output active power   Peo (pu)>"
  Bus Selector/3 -> Turbine and Excitation Regulators/2(w), [w1]  "<Rotor speed  wm  (pu)>"

== system 35 Bus Network Electricity Transmission Model/South Network/Regulators 2 ==
  m : Inport
  Bus Selector : BusSelector  OutputSignals="dq0 components.Stator voltage  vq (pu),dq0 components.Stator voltage  vd (pu),Mechanical.Rotor speed  wm  (pu),Output active power   Peo (pu)"
  Constant : Constant  Value=0.8
  Constant1 : Constant
  Math Function : Math  Operator=hypot
  Turbine and Excitation Regulators : Subsystem
  Pm : Outport
  Vf : Outport  Port=2
  tag scope: Vm2=global, w2=global
  wires:
  Constant1/1 -> Turbine and Excitation Regulators/4(Vref)
  Turbine and Excitation Regulators/1(Pm) -> Pm/1
  m/1 -> Bus Selector/1
  Turbine and Excitation Regulators/2(Vf) -> Vf/1
  Bus Selector/1 -> Math Function/1  "<Stator voltage  vq (pu)>"
  Math Function/1 -> [Vm2], Turbine and Excitation Regulators/5(Vm)
  Bus Selector/2 -> Math Function/2  "<Stator voltage  vd (pu)>"
  Constant/1 -> Turbine and Excitation Regulators/1(pref)
  Bus Selector/3 -> [w2], Turbine and Excitation Regulators/2(w)  "<Rotor speed  wm  (pu)>"
  Bus Selector/4 -> Turbine and Excitation Regulators/3(Pe 0)  "<Output active power   Peo (pu)>"

== system 35 Bus Network Electricity Transmission Model/South Network/Regulators 3 ==
  m : Inport
  Bus Selector : BusSelector  OutputSignals="dq0 components.Stator voltage  vq (pu),dq0 components.Stator voltage  vd (pu),Mechanical.Rotor speed  wm  (pu),Output active power   Peo (pu)"
  Constant : Constant  Value=0.874
  Constant1 : Constant
  Math Function : Math  Operator=hypot
  Turbine and Excitation Regulators : Subsystem
  Pm : Outport
  Vf : Outport  Port=2
  tag scope: Vm3=global, w3=global
  wires:
  Bus Selector/4 -> Turbine and Excitation Regulators/3(Pe 0)  "<Output active power   Peo (pu)>"
  Constant1/1 -> Turbine and Excitation Regulators/4(Vref)
  Bus Selector/3 -> [w3], Turbine and Excitation Regulators/2(w)  "<Rotor speed  wm  (pu)>"
  Turbine and Excitation Regulators/1(Pm) -> Pm/1
  m/1 -> Bus Selector/1
  Turbine and Excitation Regulators/2(Vf) -> Vf/1
  Bus Selector/1 -> Math Function/1  "<Stator voltage  vq (pu)>"
  Math Function/1 -> [Vm3], Turbine and Excitation Regulators/5(Vm)
  Bus Selector/2 -> Math Function/2  "<Stator voltage  vd (pu)>"
  Constant/1 -> Turbine and Excitation Regulators/1(pref)

== system 35 Bus Network Electricity Transmission Model/South Network/Regulators 4 ==
  m : Inport
  Bus Selector : BusSelector  OutputSignals="dq0 components.Stator voltage  vq (pu),dq0 components.Stator voltage  vd (pu),Mechanical.Rotor speed  wm  (pu),Output active power   Peo (pu)"
  Constant : Constant  Value=0.842
  Constant1 : Constant
  Math Function : Math  Operator=hypot
  Turbine and Excitation Regulators : Subsystem
  Pm : Outport
  Vf : Outport  Port=2
  tag scope: Vm4=global, w4=global
  wires:
  Bus Selector/4 -> Turbine and Excitation Regulators/3(Pe 0)  "<Output active power   Peo (pu)>"
  Constant1/1 -> Turbine and Excitation Regulators/4(Vref)
  Bus Selector/3 -> [w4], Turbine and Excitation Regulators/2(w)  "<Rotor speed  wm  (pu)>"
  Turbine and Excitation Regulators/1(Pm) -> Pm/1
  m/1 -> Bus Selector/1
  Turbine and Excitation Regulators/2(Vf) -> Vf/1
  Bus Selector/1 -> Math Function/1  "<Stator voltage  vq (pu)>"
  Math Function/1 -> [Vm4], Turbine and Excitation Regulators/5(Vm)
  Bus Selector/2 -> Math Function/2  "<Stator voltage  vd (pu)>"
  Constant/1 -> Turbine and Excitation Regulators/1(pref)

== system 35 Bus Network Electricity Transmission Model/South Network/Regulators 5 ==
  m : Inport
  Bus Selector : BusSelector  OutputSignals="dq0 components.Stator voltage  vq (pu),dq0 components.Stator voltage  vd (pu),Mechanical.Rotor speed  wm  (pu),Output active power   Peo (pu)"
  Constant : Constant  Value=0.881
  Constant1 : Constant
  Math Function : Math  Operator=hypot
  Turbine and Excitation Regulators : Subsystem
  Pm : Outport
  Vf : Outport  Port=2
  tag scope: Vm5=global, w5=global
  wires:
  Constant1/1 -> Turbine and Excitation Regulators/4(Vref)
  Turbine and Excitation Regulators/1(Pm) -> Pm/1
  m/1 -> Bus Selector/1
  Turbine and Excitation Regulators/2(Vf) -> Vf/1
  Math Function/1 -> [Vm5], Turbine and Excitation Regulators/5(Vm)
  Constant/1 -> Turbine and Excitation Regulators/1(pref)
  Bus Selector/1 -> Math Function/1  "<Stator voltage  vq (pu)>"
  Bus Selector/2 -> Math Function/2  "<Stator voltage  vd (pu)>"
  Bus Selector/4 -> Turbine and Excitation Regulators/3(Pe 0)  "<Output active power   Peo (pu)>"
  Bus Selector/3 -> Turbine and Excitation Regulators/2(w), [w5]  "<Rotor speed  wm  (pu)>"

== system 35 Bus Network Electricity Transmission Model/South Network/Regulators 6 ==
  m : Inport
  Bus Selector : BusSelector  OutputSignals="dq0 components.Stator voltage  vq (pu),dq0 components.Stator voltage  vd (pu),Mechanical.Rotor speed  wm  (pu),Output active power   Peo (pu)"
  Constant : Constant  Value=0.847
  Constant1 : Constant
  Math Function : Math  Operator=hypot
  Turbine and Excitation Regulators : Subsystem
  Pm : Outport
  Vf : Outport  Port=2
  tag scope: Vm6=global, w6=global
  wires:
  Constant1/1 -> Turbine and Excitation Regulators/4(Vref)
  Turbine and Excitation Regulators/1(Pm) -> Pm/1
  m/1 -> Bus Selector/1
  Turbine and Excitation Regulators/2(Vf) -> Vf/1
  Math Function/1 -> [Vm6], Turbine and Excitation Regulators/5(Vm)
  Constant/1 -> Turbine and Excitation Regulators/1(pref)
  Bus Selector/1 -> Math Function/1  "<Stator voltage  vq (pu)>"
  Bus Selector/2 -> Math Function/2  "<Stator voltage  vd (pu)>"
  Bus Selector/4 -> Turbine and Excitation Regulators/3(Pe 0)  "<Output active power   Peo (pu)>"
  Bus Selector/3 -> Turbine and Excitation Regulators/2(w), [w6]  "<Rotor speed  wm  (pu)>"

== system 35 Bus Network Electricity Transmission Model/400 kV Solar Farm/DC//DC Boost Converter/MPPT ==
  PV_Current : Inport
  PV_Voltage : Inport  Port=2
  Add : Sum  Inputs=+-
  Deblock : Step  Time=0.5  SampleTime=0
  Duty Cycle : Constant  Value=Di
  "MPPT " : Subsystem
  PWM Generator (DC-DC) : spsPWMGeneratorDCDCLib/PWM Generator (DC-DC)  Fsw=fp  Ts=Tp
  Saturation : Saturate  UpperLimit=1  LowerLimit=0
  Pulses : Outport
  tag scope: D1=global
  wires:
  "MPPT "/1(delta D) -> Add/2
  Saturation/1 -> PWM Generator (DC-DC)/1, [D1]
  PV_Voltage/1 -> "MPPT "/2(PV_Voltage)
  Add/1 -> Saturation/1
  Deblock/1 -> "MPPT "/3(Switch port)
  Duty Cycle/1 -> Add/1
  PV_Current/1 -> "MPPT "/1(PV_Current)
  PWM Generator (DC-DC)/1 -> Pulses/1

== system 35 Bus Network Electricity Transmission Model/400 kV Solar Farm/DC//DC Boost Converter/Pmean Calculation ==
  Product1 : Product
  W to KW : Gain  Gain=1/1000
  tag scope: Pmean_PV1=global
  wires:
  Product1/1 -> W to KW/1
  [Imean_PV1] -> Product1/2
  [Vmean_PV1] -> Product1/1
  W to KW/1 -> [Pmean_PV1]

== system 35 Bus Network Electricity Transmission Model/400 kV Solar Farm/DC//DC Boost Converter1/MPPT ==
  PV_Current : Inport
  PV_Voltage : Inport  Port=2
  Add : Sum  Inputs=+-
  Deblock : Step  Time=0.5  SampleTime=0
  Duty Cycle : Constant  Value=Di
  "MPPT " : Subsystem
  PWM Generator (DC-DC) : spsPWMGeneratorDCDCLib/PWM Generator (DC-DC)  Fsw=fp  Ts=Tp
  Saturation : Saturate  UpperLimit=1  LowerLimit=0
  Pulses : Outport
  tag scope: D2=global
  wires:
  "MPPT "/1(delta D) -> Add/2
  Saturation/1 -> PWM Generator (DC-DC)/1, [D2]
  PV_Voltage/1 -> "MPPT "/2(PV_Voltage)
  Add/1 -> Saturation/1
  Deblock/1 -> "MPPT "/3(Switch port)
  Duty Cycle/1 -> Add/1
  PV_Current/1 -> "MPPT "/1(PV_Current)
  PWM Generator (DC-DC)/1 -> Pulses/1

== system 35 Bus Network Electricity Transmission Model/400 kV Solar Farm/DC//DC Boost Converter1/Pmean Calculation ==
  Product1 : Product
  W to KW : Gain  Gain=1/1000
  tag scope: Pmean_PV2=global
  wires:
  Product1/1 -> W to KW/1
  [Imean_PV2] -> Product1/2
  [Vmean_PV2] -> Product1/1
  W to KW/1 -> [Pmean_PV2]

== system 35 Bus Network Electricity Transmission Model/400 kV Solar Farm/DC//DC Boost Converter2/MPPT ==
  PV_Current : Inport
  PV_Voltage : Inport  Port=2
  Add : Sum  Inputs=+-
  Deblock : Step  Time=0.5  SampleTime=0
  Duty Cycle : Constant  Value=Di
  "MPPT " : Subsystem
  PWM Generator (DC-DC) : spsPWMGeneratorDCDCLib/PWM Generator (DC-DC)  Fsw=fp  Ts=Tp
  Saturation : Saturate  UpperLimit=1  LowerLimit=0
  Pulses : Outport
  tag scope: D3=global
  wires:
  "MPPT "/1(delta D) -> Add/2
  Saturation/1 -> PWM Generator (DC-DC)/1, [D3]
  PV_Voltage/1 -> "MPPT "/2(PV_Voltage)
  Add/1 -> Saturation/1
  Deblock/1 -> "MPPT "/3(Switch port)
  Duty Cycle/1 -> Add/1
  PV_Current/1 -> "MPPT "/1(PV_Current)
  PWM Generator (DC-DC)/1 -> Pulses/1

== system 35 Bus Network Electricity Transmission Model/400 kV Solar Farm/DC//DC Boost Converter2/Pmean Calculation ==
  Product1 : Product
  W to KW : Gain  Gain=1/1000
  tag scope: Pmean_PV3=global
  wires:
  Product1/1 -> W to KW/1
  [Imean_PV3] -> Product1/2
  [Vmean_PV3] -> Product1/1
  W to KW/1 -> [Pmean_PV3]

== system 35 Bus Network Electricity Transmission Model/400 kV Solar Farm/DC//DC Boost Converter3/MPPT ==
  PV_Current : Inport
  PV_Voltage : Inport  Port=2
  Add : Sum  Inputs=+-
  Deblock : Step  Time=0.5  SampleTime=0
  Duty Cycle : Constant  Value=Di
  "MPPT " : Subsystem
  PWM Generator (DC-DC) : spsPWMGeneratorDCDCLib/PWM Generator (DC-DC)  Fsw=fp  Ts=Tp
  Saturation : Saturate  UpperLimit=1  LowerLimit=0
  Pulses : Outport
  tag scope: D4=global
  wires:
  "MPPT "/1(delta D) -> Add/2
  Saturation/1 -> PWM Generator (DC-DC)/1, [D4]
  PV_Voltage/1 -> "MPPT "/2(PV_Voltage)
  Add/1 -> Saturation/1
  Deblock/1 -> "MPPT "/3(Switch port)
  Duty Cycle/1 -> Add/1
  PV_Current/1 -> "MPPT "/1(PV_Current)
  PWM Generator (DC-DC)/1 -> Pulses/1

== system 35 Bus Network Electricity Transmission Model/400 kV Solar Farm/DC//DC Boost Converter3/Pmean Calculation ==
  Product1 : Product
  W to KW : Gain  Gain=1/1000
  tag scope: Pmean_PV4=global
  wires:
  Product1/1 -> W to KW/1
  [Imean_PV4] -> Product1/2
  [Vmean_PV4] -> Product1/1
  W to KW/1 -> [Pmean_PV4]
